simulink model "HalfCarModel"  (R2018b)
settings: Solver=VariableStepAuto  StartTime=0.0  StopTime=10  RelTol=1e-3
values from neighbouring files (symbols this model uses):
  a = 1.14    [half_parameters.m]
  b = 1.71    [half_parameters.m]
  cs_c = 15000    [half_parameters.m]    (also in parameters.m = 1000)
  cs_e = cs_c    (= 15000)    [half_parameters.m]    (also in parameters.m = 1000)
  g = 9.81    [half_parameters.m]    (also in parameters.m)
  I = 3380    [half_parameters.m]
  IC = 0    [half_parameters.m]
  ks = 15e4    (= 150000)    [half_parameters.m]    (also in parameters.m = 20000)
  ktc = 35e4    (= 350000)    [half_parameters.m]    (also in parameters.m = 140000)
  kte = ktc    (= 350000)    [half_parameters.m]    (also in parameters.m = 140000)
  m1 = 2600    [half_parameters.m]    (also in parameters.m = 250)
  m2 = 20    [half_parameters.m]    (also in parameters.m)
  v = v_kph * 1000/60^2    (= 16.6666666667)    [half_parameters.m]
  x0 = 0.2    [half_parameters.m]    (also in parameters.m)
undefined symbols (not defined in the file or in its folder): kstiff
libraries: simulink x2
settings Model: Creator=Hannah  LastModifiedBy=Hannah

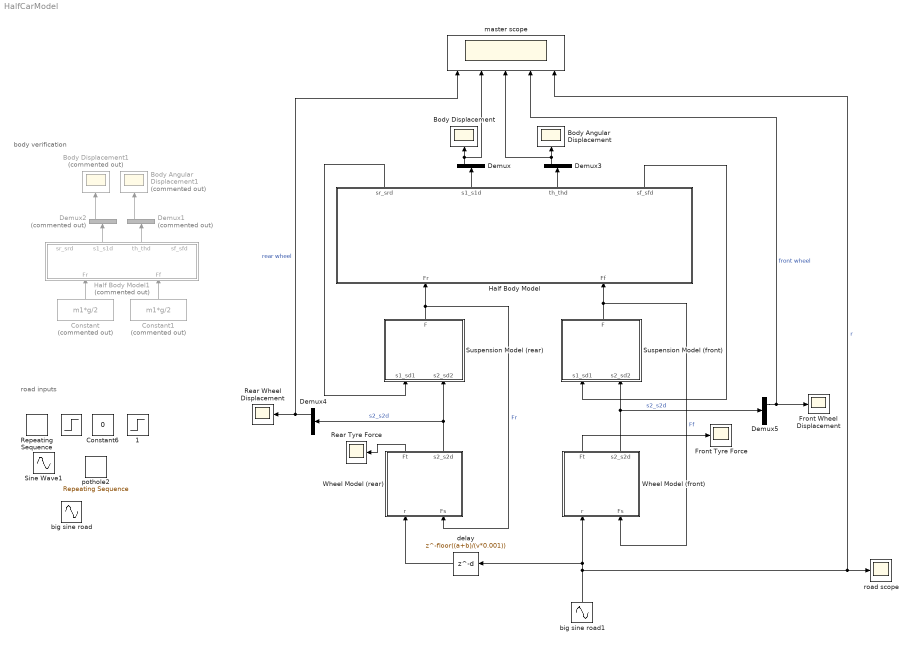
== system HalfCarModel ==
  note: body
      | verification
  note: road inputs
  " " : Step  SampleTime=0
  " 1" : Step  After=-1  SampleTime=0
  "   Front Wheel Displacement " : Scope
  Body Displacement : Scope
  Body Displacement1 : Scope  Commented=on
  Body Angular Displacement : Scope
  Body Angular Displacement1 : Scope  Commented=on
  Constant : Constant  Commented=on  Value=m1*g/2
  Constant1 : Constant  Commented=on  Value=m1*g/2
  Constant6 : Constant  Value=0
  Demux{,3..5} (4 alike) : Demux  Outputs=2
  Demux1 : Demux  Commented=on  Outputs=2
  Demux2 : Demux  Commented=on  Outputs=2
  Front Tyre Force : Scope
  Half Body Model : Subsystem
      mask Display: image("half_car_body.png")
  Half Body Model1 : Subsystem  Commented=on
      mask Display: image("half_car_body.png")
  Rear Tyre Force : Scope
  "Rear Wheel Displacement " : Scope
  Repeating Sequence : simulink/Sources/Repeating Sequence  rep_seq_t=[0 3 5 10 12 15]  rep_seq_y=[0 0 1 1 0 0]
  Sine Wave1 : Sin  Amplitude=0.1  Frequency=2*pi*v  SampleTime=0
  Suspension Model (front) : Subsystem
      mask Display: image('suspension.png')
  Suspension Model (rear) : Subsystem
      mask Display: image('suspension.png')
  Wheel Model (front) : Subsystem
      mask Display: image('wheel.png')
  Wheel Model (rear) : Subsystem
      mask Display: image('wheel.png')
  big sine road : Sin  Frequency=2*pi*v/20  SampleTime=0
  big sine road1 : Sin  Frequency=2*pi*v/20  SampleTime=0
  delay : Delay  DelayLength=floor((a+b)/(v*0.001))  SampleTime=0.001
  master scope : Scope  NumInputPorts=5
  pothole2 : simulink/Sources/Repeating Sequence  rep_seq_t=[0 5 5.2 5.8 6 10]/v  rep_seq_y=[0 0 -0.2 -0.2 0 0]
  road scope : Scope
  wires:
  Demux2/1 -> Body Displacement1/1
  Suspension Model (rear)/1(F) -> Wheel Model (rear)/2(Fs), Half Body Model/1(Fr)  "Fr"
  Suspension Model (front)/1(F) -> Wheel Model (front)/2(Fs), Half Body Model/2(Ff)  "Ff"
  big sine road1/1 -> delay/1, Wheel Model (front)/1(r), road scope/1, master scope/5  "r"
  Half Body Model/1(sr_srd) -> Suspension Model (rear)/1(s1_sd1)
  Half Body Model/4(sf_sfd) -> Suspension Model (front)/1(s1_sd1)
  Half Body Model/2(s1_s1d) -> Demux/1
  Half Body Model/3(th_thd) -> Demux3/1
  delay/1 -> Wheel Model (rear)/1(r)
  Half Body Model1/2(s1_s1d) -> Demux2/1
  Half Body Model1/3(th_thd) -> Demux1/1
  Demux1/1 -> Body Angular Displacement1/1
  Constant/1 -> Half Body Model1/1(Fr)
  Constant1/1 -> Half Body Model1/2(Ff)
  Demux/1 -> master scope/2, Body Displacement/1
  Wheel Model (rear)/1(Ft) -> Rear Tyre Force/1
  Wheel Model (front)/1(Ft) -> Front Tyre Force/1
  Demux4/1 -> master scope/1, "Rear Wheel Displacement "/1  "rear wheel"
  Wheel Model (rear)/2(s2_s2d) -> Demux4/1, Suspension Model (rear)/2(s2_sd2)  "s2_s2d"
  Demux5/1 -> "   Front Wheel Displacement "/1, master scope/4  "front wheel"
  Wheel Model (front)/2(s2_s2d) -> Demux5/1, Suspension Model (front)/2(s2_sd2)  "s2_s2d"
  Demux3/1 -> master scope/3, Body Angular Displacement/1

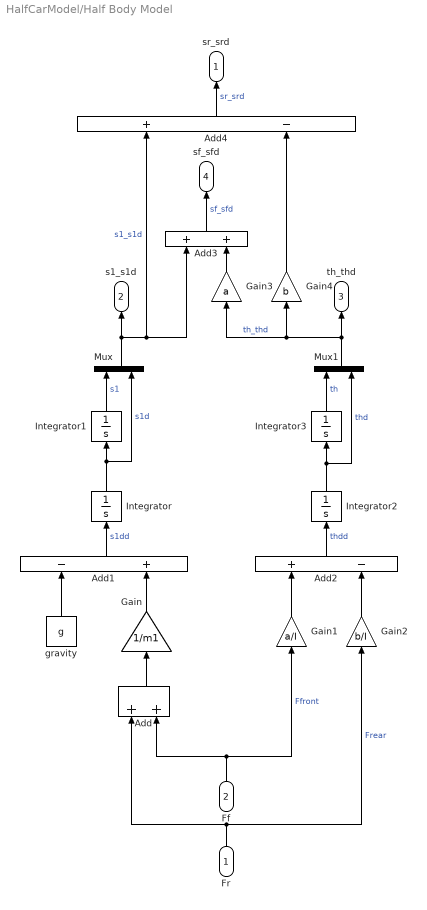
== system HalfCarModel/Half Body Model ==
  Fr : Inport
  Ff : Inport  Port=2
  Add : Sum
  Add1 : Sum  Inputs=-+
  Add2 : Sum  Inputs=+-
  Add3 : Sum
  Add4 : Sum  Inputs=+-
  Gain : Gain  Gain=1/m1
  Gain1 : Gain  Gain=a/I
  Gain2 : Gain  Gain=b/I
  Gain3 : Gain  Gain=a
  Gain4 : Gain  Gain=b
  Integrator : Integrator
  Integrator1 : Integrator  InitialCondition=IC
  Integrator2 : Integrator
  Integrator3 : Integrator
  Mux : Mux  Inputs=2
  Mux1 : Mux  Inputs=2
  "gravity " : Constant  Value=g
  sr_srd : Outport
  s1_s1d : Outport  Port=2
  th_thd : Outport  Port=3
  sf_sfd : Outport  Port=4
  wires:
  Fr/1 -> Add/1, Gain2/1  "Frear"
  Ff/1 -> Add/2, Gain1/1  "Ffront"
  Add/1 -> Gain/1
  Gain/1 -> Add1/2
  "gravity "/1 -> Add1/1
  Add1/1 -> Integrator/1  "s1dd"
  Integrator/1 -> Mux/2, Integrator1/1  "s1d"
  Integrator1/1 -> Mux/1  "s1"
  Mux/1 -> Add3/1, Add4/1, s1_s1d/1  "s1_s1d"
  Gain1/1 -> Add2/1
  Gain2/1 -> Add2/2
  Add2/1 -> Integrator2/1  "thdd"
  Integrator2/1 -> Mux1/2, Integrator3/1  "thd"
  Integrator3/1 -> Mux1/1  "th"
  Mux1/1 -> Gain3/1, Gain4/1, th_thd/1  "th_thd"
  Gain3/1 -> Add3/2
  Add3/1 -> sf_sfd/1  "sf_sfd"
  Add4/1 -> sr_srd/1  "sr_srd"
  Gain4/1 -> Add4/2

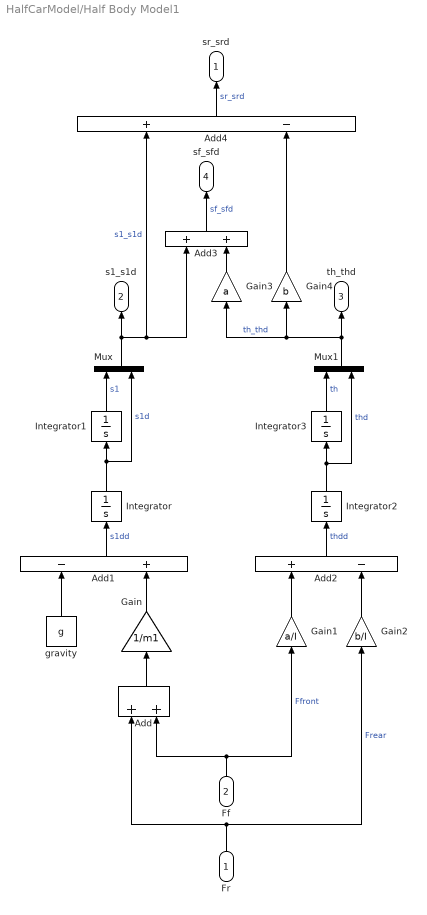
== system HalfCarModel/Half Body Model1 ==
  Fr : Inport
  Ff : Inport  Port=2
  Add : Sum
  Add1 : Sum  Inputs=-+
  Add2 : Sum  Inputs=+-
  Add3 : Sum
  Add4 : Sum  Inputs=+-
  Gain : Gain  Gain=1/m1
  Gain1 : Gain  Gain=a/I
  Gain2 : Gain  Gain=b/I
  Gain3 : Gain  Gain=a
  Gain4 : Gain  Gain=b
  Integrator{,1..3} (4 alike) : Integrator
  Mux : Mux  Inputs=2
  Mux1 : Mux  Inputs=2
  "gravity " : Constant  Value=g
  sr_srd : Outport
  s1_s1d : Outport  Port=2
  th_thd : Outport  Port=3
  sf_sfd : Outport  Port=4
  wires:
  Fr/1 -> Add/1, Gain2/1  "Frear"
  Ff/1 -> Add/2, Gain1/1  "Ffront"
  Add/1 -> Gain/1
  Gain/1 -> Add1/2
  "gravity "/1 -> Add1/1
  Add1/1 -> Integrator/1  "s1dd"
  Integrator/1 -> Mux/2, Integrator1/1  "s1d"
  Integrator1/1 -> Mux/1  "s1"
  Mux/1 -> Add3/1, Add4/1, s1_s1d/1  "s1_s1d"
  Gain1/1 -> Add2/1
  Gain2/1 -> Add2/2
  Add2/1 -> Integrator2/1  "thdd"
  Integrator2/1 -> Mux1/2, Integrator3/1  "thd"
  Integrator3/1 -> Mux1/1  "th"
  Mux1/1 -> Gain3/1, Gain4/1, th_thd/1  "th_thd"
  Gain3/1 -> Add3/2
  Add3/1 -> sf_sfd/1  "sf_sfd"
  Add4/1 -> sr_srd/1  "sr_srd"
  Gain4/1 -> Add4/2

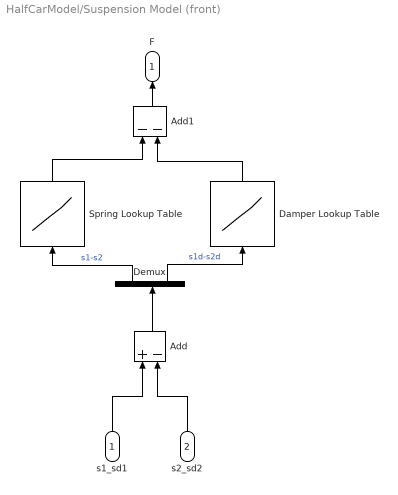
== system HalfCarModel/Suspension Model (front) ==
  s1_sd1 : Inport
  s2_sd2 : Inport  Port=2
  Add : Sum  Inputs=+-
  Add1 : Sum  Inputs=--
  Damper Lookup Table : Lookup_n-D  NumberOfTableDimensions=1  BreakpointsForDimension1=[-1 0 1]  Table=[-cs_c, 0, cs_e]  InternalRulePriority=Speed  RndMeth=Simplest  InputSameDT=on
  Demux : Demux  Outputs=2
  Spring Lookup Table : Lookup_n-D  NumberOfTableDimensions=1  BreakpointsForDimension1=[-2*x0, -x0, x0, 2*x0]  Table=[-(ks+kstiff)*x0, -ks*x0, ks*x0, (ks+kstiff)*x0]  InternalRulePriority=Speed  RndMeth=Simplest  InputSameDT=on
  F : Outport
  wires:
  s2_sd2/1 -> Add/2
  Spring Lookup Table/1 -> Add1/1
  Add1/1 -> F/1
  Damper Lookup Table/1 -> Add1/2
  Demux/2 -> Damper Lookup Table/1  "s1d-s2d"
  Demux/1 -> Spring Lookup Table/1  "s1-s2"
  Add/1 -> Demux/1
  s1_sd1/1 -> Add/1

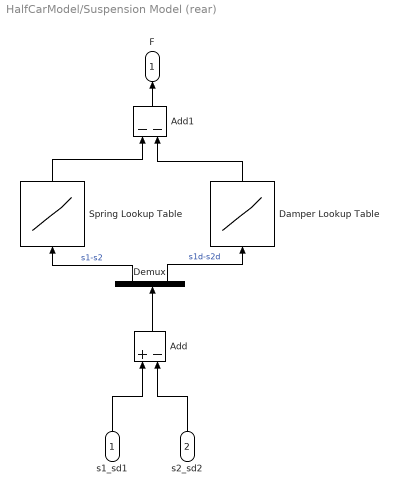
== system HalfCarModel/Suspension Model (rear) ==
  s1_sd1 : Inport
  s2_sd2 : Inport  Port=2
  Add : Sum  Inputs=+-
  Add1 : Sum  Inputs=--
  Damper Lookup Table : Lookup_n-D  NumberOfTableDimensions=1  BreakpointsForDimension1=[-1 0 1]  Table=[-cs_c, 0, cs_e]  InternalRulePriority=Speed  RndMeth=Simplest  InputSameDT=on
  Demux : Demux  Outputs=2
  Spring Lookup Table : Lookup_n-D  NumberOfTableDimensions=1  BreakpointsForDimension1=[-2*x0, -x0, x0, 2*x0]  Table=[-(ks+kstiff)*x0, -ks*x0, ks*x0, (ks+kstiff)*x0]  InternalRulePriority=Speed  RndMeth=Simplest  InputSameDT=on
  F : Outport
  wires:
  s2_sd2/1 -> Add/2
  Spring Lookup Table/1 -> Add1/1
  Add1/1 -> F/1
  Damper Lookup Table/1 -> Add1/2
  Demux/2 -> Damper Lookup Table/1  "s1d-s2d"
  Demux/1 -> Spring Lookup Table/1  "s1-s2"
  Add/1 -> Demux/1
  s1_sd1/1 -> Add/1

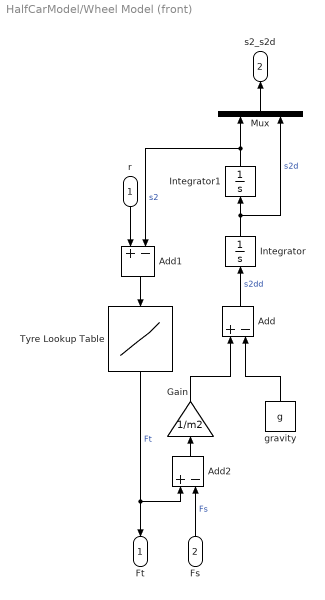
== system HalfCarModel/Wheel Model (front) ==
  r : Inport
  Fs : Inport  Port=2
  Add : Sum  Inputs=+-
  Add1 : Sum  Inputs=+-
  Add2 : Sum  Inputs=+-
  Gain : Gain  Gain=1/m2
  Integrator : Integrator
  Integrator1 : Integrator  InitialCondition=IC
  Mux : Mux  Inputs=2
  Tyre Lookup Table : Lookup_n-D  NumberOfTableDimensions=1  BreakpointsForDimension1=[-1 0 1]  Table=[-kte, 0, ktc]  InternalRulePriority=Speed  RndMeth=Simplest  InputSameDT=on
  gravity : Constant  Value=g
  Ft : Outport
  s2_s2d : Outport  Port=2
  wires:
  r/1 -> Add1/1
  Fs/1 -> Add2/2  "Fs"
  Add2/1 -> Gain/1
  Gain/1 -> Add/1
  Integrator/1 -> Mux/2, Integrator1/1  "s2d"
  Add/1 -> Integrator/1  "s2dd"
  Tyre Lookup Table/1 -> Ft/1, Add2/1  "Ft"
  gravity/1 -> Add/2
  Integrator1/1 -> Add1/2, Mux/1  "s2"
  Add1/1 -> Tyre Lookup Table/1
  Mux/1 -> s2_s2d/1

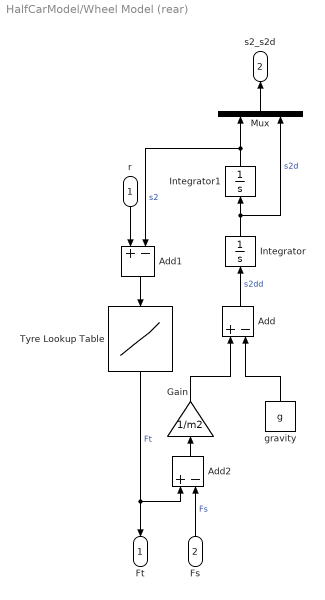
== system HalfCarModel/Wheel Model (rear) ==
  r : Inport
  Fs : Inport  Port=2
  Add : Sum  Inputs=+-
  Add1 : Sum  Inputs=+-
  Add2 : Sum  Inputs=+-
  Gain : Gain  Gain=1/m2
  Integrator : Integrator
  Integrator1 : Integrator  InitialCondition=IC
  Mux : Mux  Inputs=2
  Tyre Lookup Table : Lookup_n-D  NumberOfTableDimensions=1  BreakpointsForDimension1=[-1 0 1]  Table=[-kte, 0, ktc]  InternalRulePriority=Speed  RndMeth=Simplest  InputSameDT=on
  gravity : Constant  Value=g
  Ft : Outport
  s2_s2d : Outport  Port=2
  wires:
  r/1 -> Add1/1
  Fs/1 -> Add2/2  "Fs"
  Add2/1 -> Gain/1
  Gain/1 -> Add/1
  Integrator/1 -> Mux/2, Integrator1/1  "s2d"
  Add/1 -> Integrator/1  "s2dd"
  Tyre Lookup Table/1 -> Ft/1, Add2/1  "Ft"
  gravity/1 -> Add/2
  Integrator1/1 -> Add1/2, Mux/1  "s2"
  Add1/1 -> Tyre Lookup Table/1
  Mux/1 -> s2_s2d/1
